simulink model "psex"  (Simulink 8.5)
settings: Solver=ode45  SolverMode=SingleTasking  StartTime=0.0  StopTime=1  RelTol=1e-3  AbsTol=1e-6
libraries: elements x13, inputs x2
settings Model: Creator=PC  LastModifiedBy=PC
settings DataIOCC: LimitDataPoints=off
settings OptimizationCC: BlockReduction=off  BooleanDataType=off  ExpressionDepthLimit=128
settings DebuggingCC: SaveWithParameterizedLinksMsg=none  SignalResolutionControl=TryResolveAllWithWarning  MultiTaskDSMMsg=warning  MultiTaskCondExecSysMsg=none  FcnCallInpInsideContextMsg=EnableAllAsError  StateNameClashWarn=none  StrictBusMsg=None
settings HardwareCC: TargetUnknown=on
settings RTWCC: TemplateMakefile=grt_vc.tmf

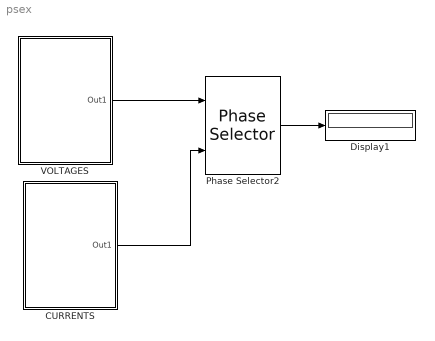
== system psex ==
  CURRENTS : Subsystem
      mask Display: disp('Orthogonal \ncomponents\n of phase\n currents' )
  Display1 : Display
  Phase Selector2 : elements/Phase Selector  THI=3  THV=3  THZ=3  THG=0.5  METHOD=Current and Voltage and Impedance
  VOLTAGES : Subsystem
      mask Display: disp('Orthogonal \ncomponents\n of phase\n voltages' )
  wires:
  Phase Selector2/1 -> Display1/1
  VOLTAGES/1(Out1) -> Phase Selector2/1
  CURRENTS/1(Out1) -> Phase Selector2/2

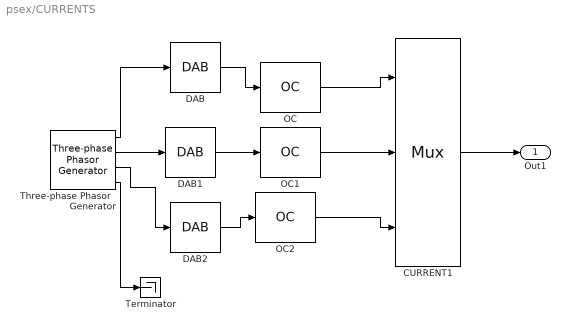
== system psex/CURRENTS ==
  CURRENT1 : Mux  Inputs=3
  DAB : elements/DAB  filter=on  approx=Bessel  order=2  numerator=[]  denominator=[]  freq=180  resdis=on  vertres=12  xmax=10  winsize=40  G=1.0  fs=60*40
  DAB1 : elements/DAB  filter=on  approx=Bessel  order=2  numerator=[]  denominator=[]  freq=180  resdis=on  vertres=12  xmax=10  winsize=40  G=1.0  fs=60*40
  DAB2 : elements/DAB  filter=on  approx=Bessel  order=2  numerator=[]  denominator=[]  freq=180  resdis=on  vertres=12  xmax=10  winsize=40  G=1.0  fs=60*40
  OC : elements/OC  tfilt=Fourier  rfilt=[ ]  ifilt=[ ]  tlen=full  N1=40
  OC1 : elements/OC  tfilt=Fourier  rfilt=[ ]  ifilt=[ ]  tlen=full  N1=40
  OC2 : elements/OC  tfilt=Fourier  rfilt=[ ]  ifilt=[ ]  tlen=full  N1=40
  Terminator : Terminator
  Three-phase Phasor   Generator : inputs/Three-phase Phasor   Generator  phase_type=Phase quantities-unsymmetrical  phase1=[2 0]  phase2=[2 0]  phase3=[7 0]  f=60  to=0
  Out1 : Outport
  wires:
  CURRENT1/1 -> Out1/1
  OC2/1 -> CURRENT1/3
  OC1/1 -> CURRENT1/2
  OC/1 -> CURRENT1/1
  DAB/1 -> OC/1
  DAB1/1 -> OC1/1
  DAB2/1 -> OC2/1
  Three-phase Phasor   Generator/4 -> Terminator/1
  Three-phase Phasor   Generator/1 -> DAB/1
  Three-phase Phasor   Generator/2 -> DAB1/1
  Three-phase Phasor   Generator/3 -> DAB2/1

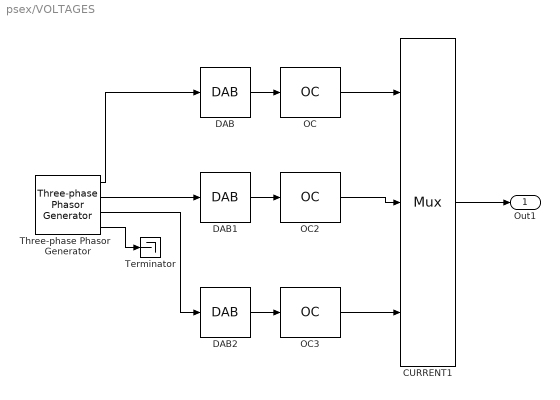
== system psex/VOLTAGES ==
  CURRENT1 : Mux  Inputs=3
  DAB : elements/DAB  filter=on  approx=Bessel  order=2  numerator=[]  denominator=[]  freq=180  resdis=on  vertres=12  xmax=10  winsize=40  G=1.0  fs=60*40
  DAB1 : elements/DAB  filter=on  approx=Bessel  order=2  numerator=[]  denominator=[]  freq=180  resdis=on  vertres=12  xmax=10  winsize=40  G=1.0  fs=60*40
  DAB2 : elements/DAB  filter=on  approx=Bessel  order=2  numerator=[]  denominator=[]  freq=180  resdis=on  vertres=12  xmax=10  winsize=40  G=1.0  fs=60*40
  OC : elements/OC  tfilt=Fourier  rfilt=[ ]  ifilt=[ ]  tlen=full  N1=40
  OC2 : elements/OC  tfilt=Fourier  rfilt=[ ]  ifilt=[ ]  tlen=full  N1=40
  OC3 : elements/OC  tfilt=Fourier  rfilt=[ ]  ifilt=[ ]  tlen=full  N1=40
  Terminator : Terminator
  Three-phase Phasor   Generator : inputs/Three-phase Phasor   Generator  phase_type=Phase quantities-unsymmetrical  phase1=[4 0]  phase2=[4 180]  phase3=[2 180]  f=60  to=0
  Out1 : Outport
  wires:
  Three-phase Phasor   Generator/4 -> Terminator/1
  OC/1 -> CURRENT1/1
  CURRENT1/1 -> Out1/1
  DAB/1 -> OC/1
  Three-phase Phasor   Generator/1 -> DAB/1
  DAB2/1 -> OC3/1
  OC3/1 -> CURRENT1/3
  DAB1/1 -> OC2/1
  OC2/1 -> CURRENT1/2
  Three-phase Phasor   Generator/2 -> DAB1/1
  Three-phase Phasor   Generator/3 -> DAB2/1
